simulink model "sgMdl_IO751_IO752_PROFINETSynchronous"  (R2024b)
settings: Solver=FixedStepAuto  StartTime=0.0  StopTime=inf  RelTol=1e-3  EnableMultiTasking=on
undefined symbols (not defined in the file): C
libraries: slrealtimeutilitieslib x26, simulink x3, speedgoatlib_IO751 x3, speedgoatlib_IO752 x3, speedgoatlib_interrupt x2
Description:
  | IO751 & IO752 - Synchronous PROFINET
settings Model: ModifiedByFormat=Speedgoat  Creator=Speedgoat  LastModifiedBy=Speedgoat
settings SolverCC: ConcurrentTasks=on  AlgebraicLoopSolver=TrustRegion  PositivePriorityOrder=on  AutoInsertRateTranBlk=on  InsertRTBMode=Never (minimum delay)
settings DataIOCC: SaveFormat=Array  SaveState=on  SignalLoggingName=logsOut
settings OptimizationCC: BlockReduction=off  BooleanDataType=off  OptimizeBlockIOStorage=off  BufferReuse=off  ReuseModelBlockBuffer=off  GlobalBufferReuse=off  ExpressionFolding=off  LocalBlockOutputs=off  InitFltsAndDblsToZero=on  OptimizeDataStoreBuffers=off  BusAssignmentInplaceUpdate=off
settings DebuggingCC: SaveWithParameterizedLinksMsg=none  UnderspecifiedInitializationDetection=Classic  MergeDetectMultiDrivingBlocksExec=none  CheckExecutionContextPreStartOutputMsg=on  SignalResolutionControl=TryResolveAllWithWarning  TasksWithSamePriorityMsg=none  UnconnectedInputMsg=warning  UnconnectedOutputMsg=warning  UnconnectedLineMsg=warning  SFUnexpectedBacktrackingDiag=warning  SFNoUnconditionalDefaultTransitionDiag=warning  SFExecutionAtInitializationDiag=none  ArithmeticOperatorsInVariantConditions=warning
settings HardwareCC: ProdBitPerLong=64  ProdLongLongMode=on  ProdHWDeviceType=Intel->x86-64 (Linux 64)
settings ModelReferenceCC: EnableRefExpFcnMdlSchedulingChecks=on  PropagateSignalLabelsOutOfModel=off
settings SFSimCC: SimUseLocalCustomCode=off  SimTargetLang=C++
settings RTWCC: Description=Speedgoat Real-Time Target Machine  SystemTargetFile=speedgoat.tlc  TemplateMakefile=slrealtime_default_tmf  RTWUseLocalCustomCode=off  Toolchain=Simulink Real-Time Toolchain  BuildConfiguration=Faster Runs  TargetLang=C++  GPUComputeCapability=3.5  DLArmComputeVersion=19.05
settings CodeAppCC: StateflowObjectComments=on
settings SimulinkRealTimeTargetCC: SubcomponentCodeInterfacePackaging=Reusable function  InstructionSetFMA=off  LogToMDFFile=off  SLRTFileLogMaxRuns=10
settings ConfigComp: CovMetricSettings=dw  CovSaveCumulativeToWorkspaceVar=on  CovSaveSingleToWorkspaceVar=on  CovExternalEMLEnable=off  CovSFcnEnable=off  CovBoundaryAbsTol=1.0e-5

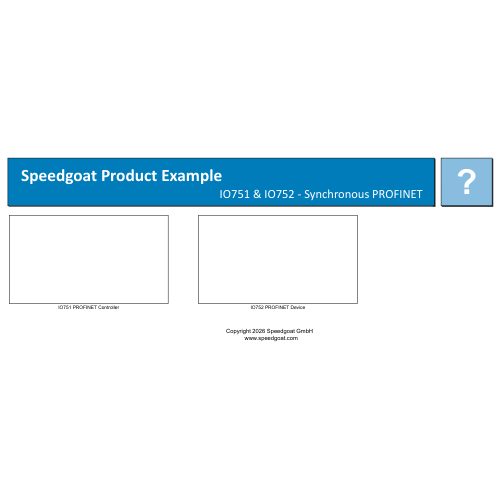
[thumbnail: Simulink's stored preview of the top-level diagram]
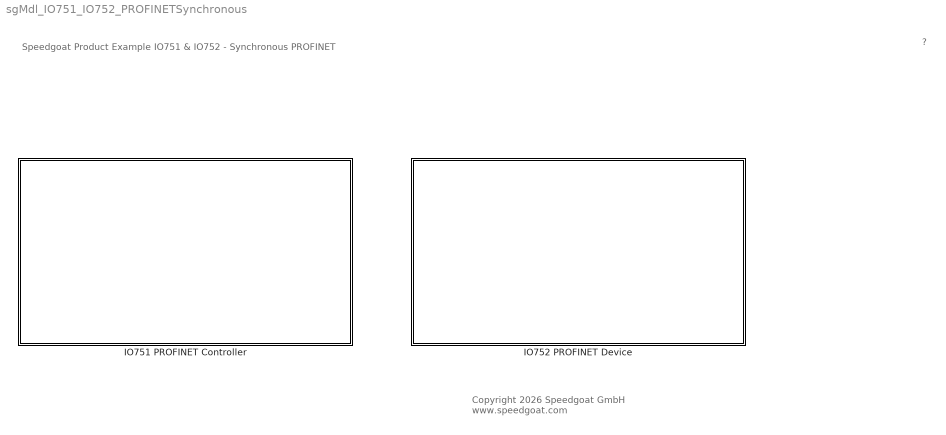
== system sgMdl_IO751_IO752_PROFINETSynchronous ==
  note: Speedgoat Product Example
      | IO751 & IO752 - Synchronous PROFINET
  note: ?
  note: Copyright 2026 Speedgoat GmbH
      |  www.speedgoat.com
  IO751 PROFINET Controller : Subsystem
  IO752 PROFINET Device : Subsystem

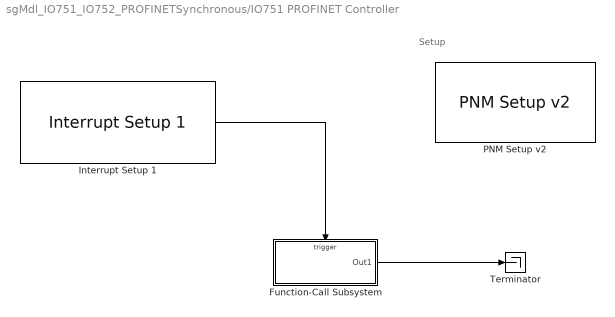
== system sgMdl_IO751_IO752_PROFINETSynchronous/IO751 PROFINET Controller ==
  note: Setup
  Function-Call Subsystem : Subsystem  TreatAsAtomicUnit=on
  Interrupt Setup 1 : speedgoatlib_interrupt/Interrupt Setup 1  parModuleTrigger=off  parPollingMode=off  parPriorityConf=High  parPriority=241  confStartFcn=IO75x_start_public  confStopFcn=IO75x_stop_public  confIsrFcn=IO75x_isr_public  confMapFcn=IO75x_map_public  confHookFile=io75x_int_hooks.c  confIrqNr=-1  confIsPolling=off  confModID=985345  confSelectedInt=Speedgoat IO75x interrupt  confSelectedId=1  confSelectedChannel=[]  confData=[]  confForcePollingMode=off
  "PNM Setup v2 " : speedgoatlib_IO751/PNM Setup v2   id=1  driveLetter=C:  configurationMode=Configuration file  mode=Polling mode  pciSlot=[9,15]  quantityOfAcyclicObjects=0  qtyMods=[1,0,0]  ConfigFile=which('IO751_IO752_Synchronous_m.nxd')  parOptAcyclic=off  protocol=IO751  firmware=PROFINET Controller
      settings: SourceProductName=IO751 PROFINET Controller
  Terminator : Terminator
  wires:
  Interrupt Setup 1/1 -> Function-Call Subsystem/Trigger
  Function-Call Subsystem/1(Out1) -> Terminator/1

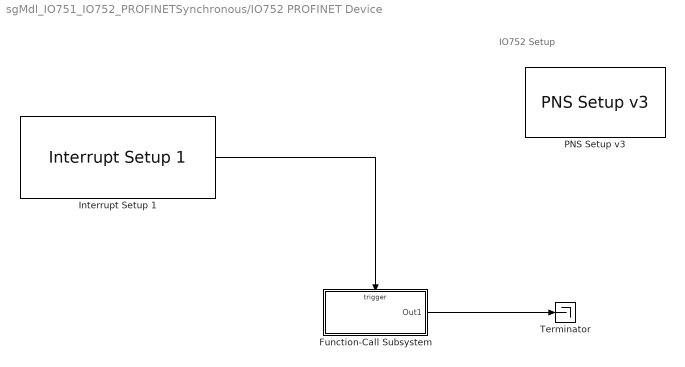
== system sgMdl_IO751_IO752_PROFINETSynchronous/IO752 PROFINET Device ==
  note: IO752 Setup
  Function-Call Subsystem : Subsystem  TreatAsAtomicUnit=on
  Interrupt Setup 1 : speedgoatlib_interrupt/Interrupt Setup 1  parModuleTrigger=off  parPollingMode=off  parPriorityConf=High  parPriority=241  confStartFcn=IO75x_start_public  confStopFcn=IO75x_stop_public  confIsrFcn=IO75x_isr_public  confMapFcn=IO75x_map_public  confHookFile=io75x_int_hooks.c  confIrqNr=-1  confIsPolling=off  confModID=919810  confSelectedInt=Speedgoat IO75x interrupt  confSelectedId=2  confSelectedChannel=[]  confData=[]  confForcePollingMode=off
  PNS Setup v3 : speedgoatlib_IO752/PNS Setup v3  id=2  PciSlot=[9,14]  StationName='cifxrepns'  BusStart=On model start  SystemRedundancy=off  RecordSuccess=on  GsdFile=[speedgoatroot, '\sg_blocks\cifx\eds\GSDML-V2.33-HILSCHER-CIFX RE PNS-20170919.xml']  VendorId=286  DeviceId=259  OptionalIdentity=off  DeviceType='cifxrepns'  OrderId='1250.1'  HwRev=2  SwRevPrefix='V'  SwRev=[3,0,0]  SerialNumber='0'  ModuleConfigTable="{ '0', '', 'CIFX RE/PNS V3.5.35 - V3.x', '8321', '', '', 'DIM 24', '', '', '0', '1', ''; '0', '1', '  CIFX RE/PNS V3.5.35 - V3.x', '8321', '8320', '', 'DIM 24', '1', '', '', '', ''; '0', '32768', '  PN-IO', '8321', '8321', '', 'DIM 24 Interfacesubmodule', '1', '', '', '', ''; '0', '32769', '  Port 1', '8321', '8322', '', 'DIM 24 Portsubmodule 1', '1', '', '', '', ''; '0', '32770', '  Port 2', '8321', '8323', '', 'DIM 24 Portsubmodule 2', '1', '', '', '', ''; '1', '', '4 Bytes Input', '8', '', '', '4byteinput', '0', '', '', '', ''; '1', '1', '  4 Bytes Input', '8', '7', '', '4byteinput', '1', '{\"Inputs\",[3],[4]}', '', '', ''; '2', '', '4 Bytes Output', '9', '', '', '4byteoutput', '0', '', '', '', ''; '2', '1', '  4 Bytes Output', '9', '8', '', '4byteoutput', '1', '', '{\"Outputs\",[3],[4]}', '', '' }"
      settings: SourceProductName=IO752 PROFINET Device
  Terminator : Terminator
  wires:
  Interrupt Setup 1/1 -> Function-Call Subsystem/Trigger
  Function-Call Subsystem/1(Out1) -> Terminator/1

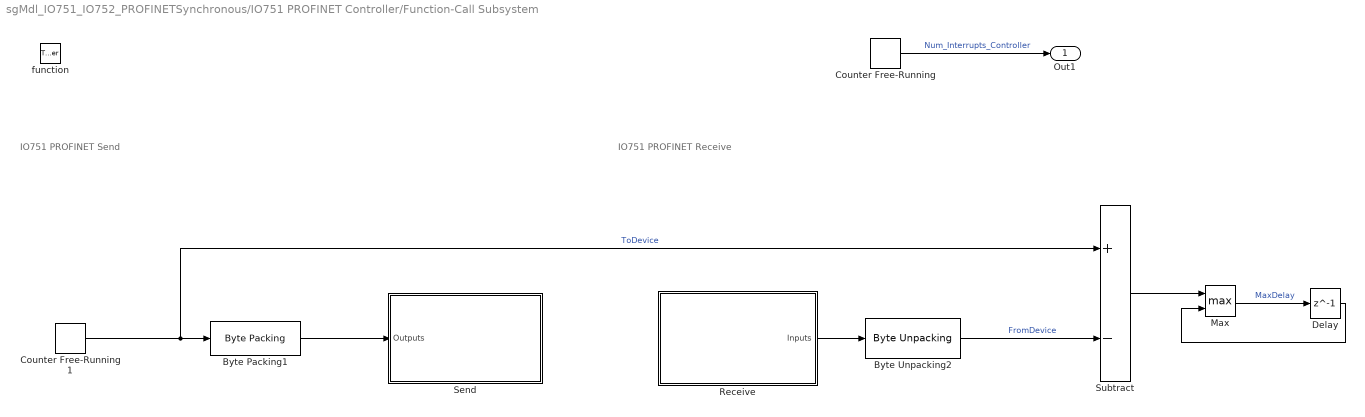
== system sgMdl_IO751_IO752_PROFINETSynchronous/IO751 PROFINET Controller/Function-Call Subsystem ==
  note: IO751 PROFINET Receive
  note: IO751 PROFINET Send
  function : TriggerPort  TriggerType=function-call  VariantControl=(inherit)
  Byte Packing1 : slrealtimeutilitieslib/Byte Packing  MaskPackedDataType=uint8  MaskUnpackedDataTypes={'uint32'}  MaskAlignment=1
  Byte Unpacking2 : slrealtimeutilitieslib/Byte Unpacking  MaskUnpackedDataTypes={'uint32'}  MaskUnpackedDataSizes={[1]}  MaskAlignment=1
  Counter Free-Running : simulink/Sources/Counter Free-Running  NumBits=16  tsamp=-1
  Counter Free-Running1 : simulink/Sources/Counter Free-Running  NumBits=32  tsamp=-1
  Delay : Delay  DelayLength=1
  Max : MinMax  Function=max  Inputs=2
  Receive : Subsystem
  Send : Subsystem
  Subtract : Sum  Inputs=+-
  Out1 : Outport
  wires:
  Counter Free-Running/1 -> Out1/1  "Num_Interrupts_Controller"
  Max/1 -> Delay/1  "MaxDelay"
  Delay/1 -> Max/2
  Counter Free-Running1/1 -> Subtract/1, Byte Packing1/1  "ToDevice"
  Subtract/1 -> Max/1
  Byte Packing1/1 -> Send/1(Outputs)
  Receive/1(Inputs) -> Byte Unpacking2/1
  Byte Unpacking2/1 -> Subtract/2  "FromDevice"

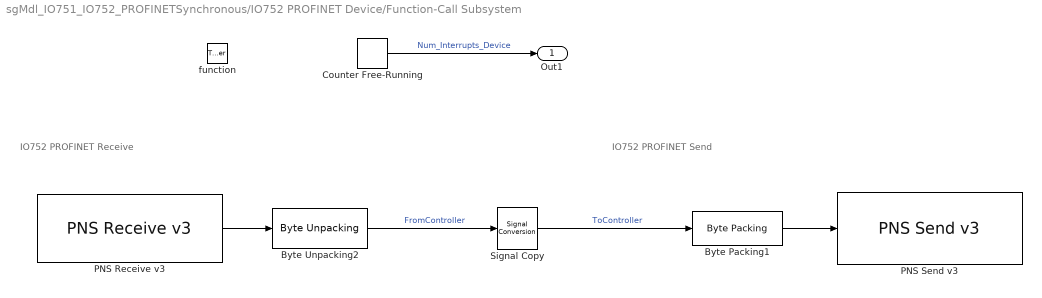
== system sgMdl_IO751_IO752_PROFINETSynchronous/IO752 PROFINET Device/Function-Call Subsystem ==
  note: IO752 PROFINET Receive
  note: IO752 PROFINET Send
  function : TriggerPort  TriggerType=function-call  VariantControl=(inherit)
  Byte Packing1 : slrealtimeutilitieslib/Byte Packing  MaskPackedDataType=uint8  MaskUnpackedDataTypes={'uint32'}  MaskAlignment=1
  Byte Unpacking2 : slrealtimeutilitieslib/Byte Unpacking  MaskUnpackedDataTypes={'uint32'}  MaskUnpackedDataSizes={[1]}  MaskAlignment=1
  Counter Free-Running : simulink/Sources/Counter Free-Running  NumBits=16  tsamp=-1
  PNS Receive v3 : speedgoatlib_IO752/PNS Receive v3  id=2  SampleTime=-1  DataLevel=Data Item  GroupDataItems=off  PortLabel1=off  PortLabel2=on  PortLabel3=off  PnModuleConfig="{ '0', '', 'CIFX RE/PNS V3.5.35 - V3.x', '8321', '', '', 'DIM 24', '', '', '0', '1', ''; '0', '1', '  CIFX RE/PNS V3.5.35 - V3.x', '8321', '8320', '', 'DIM 24', '1', '', '', '', ''; '0', '32768', '  PN-IO', '8321', '8321', '', 'DIM 24 Interfacesubmodule', '1', '', '', '', ''; '0', '32769', '  Port 1', '8321', '8322', '', 'DIM 24 Portsubmodule 1', '1', '', '', '', ''; '0', '32770', '  Port 2', '8321', '8323', '', 'DIM 24 Portsubmodule 2', '1', '', '', '', ''; '1', '', '4 Bytes Input', '8', '', '', '4byteinput', '0', '', '', '', ''; '1', '1', '  4 Bytes Input', '8', '7', '', '4byteinput', '1', '{\"Inputs\",[3],[4]}', '', '', ''; '2', '', '4 Bytes Output', '9', '', '', '4byteoutput', '0', '', '', '', ''; '2', '1', '  4 Bytes Output', '9', '8', '', '4byteoutput', '1', '', '{\"Outputs\",[3],[4]}', '', '' }"
      settings: SourceProductName=IO752 PROFINET Device
  PNS Send v3 : speedgoatlib_IO752/PNS Send v3  id=2  SampleTime=-1  DataLevel=Data Item  GroupDataItems=off  PortLabel1=off  PortLabel2=on  PortLabel3=off  PnModuleConfig="{ '0', '', 'CIFX RE/PNS V3.5.35 - V3.x', '8321', '', '', 'DIM 24', '', '', '0', '1', ''; '0', '1', '  CIFX RE/PNS V3.5.35 - V3.x', '8321', '8320', '', 'DIM 24', '1', '', '', '', ''; '0', '32768', '  PN-IO', '8321', '8321', '', 'DIM 24 Interfacesubmodule', '1', '', '', '', ''; '0', '32769', '  Port 1', '8321', '8322', '', 'DIM 24 Portsubmodule 1', '1', '', '', '', ''; '0', '32770', '  Port 2', '8321', '8323', '', 'DIM 24 Portsubmodule 2', '1', '', '', '', ''; '1', '', '4 Bytes Input', '8', '', '', '4byteinput', '0', '', '', '', ''; '1', '1', '  4 Bytes Input', '8', '7', '', '4byteinput', '1', '{\"Inputs\",[3],[4]}', '', '', ''; '2', '', '4 Bytes Output', '9', '', '', '4byteoutput', '0', '', '', '', ''; '2', '1', '  4 Bytes Output', '9', '8', '', '4byteoutput', '1', '', '{\"Outputs\",[3],[4]}', '', '' }"
      settings: SourceProductName=IO752 PROFINET Device
  Signal Copy : SignalConversion  OverrideOpt=off
  Out1 : Outport
  wires:
  PNS Receive v3/1 -> Byte Unpacking2/1
  Counter Free-Running/1 -> Out1/1  "Num_Interrupts_Device"
  Signal Copy/1 -> Byte Packing1/1  "ToController"
  Byte Unpacking2/1 -> Signal Copy/1  "FromController"
  Byte Packing1/1 -> PNS Send v3/1

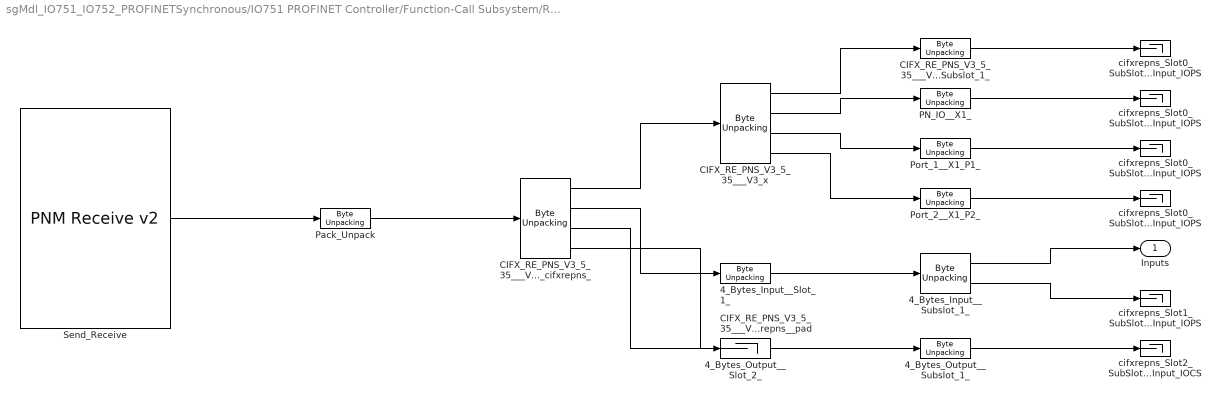
== system sgMdl_IO751_IO752_PROFINETSynchronous/IO751 PROFINET Controller/Function-Call Subsystem/Receive ==
  4_Bytes_Input__Slot_1_ : slrealtimeutilitieslib/Byte Unpacking  MaskUnpackedDataTypes={'uint8'}  MaskUnpackedDataSizes={[5]}  MaskAlignment=1
  4_Bytes_Input__Subslot_1_ : slrealtimeutilitieslib/Byte Unpacking  MaskUnpackedDataTypes={'uint8','uint8'}  MaskUnpackedDataSizes={[4],[1]}  MaskAlignment=1
  4_Bytes_Output__Slot_2_ : slrealtimeutilitieslib/Byte Unpacking  MaskUnpackedDataTypes={'uint8'}  MaskUnpackedDataSizes={[1]}  MaskAlignment=1
  4_Bytes_Output__Subslot_1_ : slrealtimeutilitieslib/Byte Unpacking  MaskUnpackedDataTypes={'uint8'}  MaskUnpackedDataSizes={[1]}  MaskAlignment=1
  CIFX_RE_PNS_V3_5_35___V3_x : slrealtimeutilitieslib/Byte Unpacking  MaskUnpackedDataTypes={'uint8','uint8','uint8','uint8'}  MaskUnpackedDataSizes={[1],[1],[1],[1]}  MaskAlignment=1
  CIFX_RE_PNS_V3_5_35___V3_x_CIFX_RE_PNS_V3_5_35___V3_x__cifxrepns_ : slrealtimeutilitieslib/Byte Unpacking  MaskUnpackedDataTypes={'uint8','uint8','uint8','uint8'}  MaskUnpackedDataSizes={[4],[5],[1],[2]}  MaskAlignment=1
  CIFX_RE_PNS_V3_5_35___V3_x_CIFX_RE_PNS_V3_5_35___V3_x__cifxrepns__pad : Terminator
  CIFX_RE_PNS_V3_5_35___V3_x__Subslot_1_ : slrealtimeutilitieslib/Byte Unpacking  MaskUnpackedDataTypes={'uint8'}  MaskUnpackedDataSizes={[1]}  MaskAlignment=1
  PN_IO__X1_ : slrealtimeutilitieslib/Byte Unpacking  MaskUnpackedDataTypes={'uint8'}  MaskUnpackedDataSizes={[1]}  MaskAlignment=1
  Pack_Unpack : slrealtimeutilitieslib/Byte Unpacking  MaskUnpackedDataTypes={'uint8'}  MaskUnpackedDataSizes={[12]}  MaskAlignment=1
  Port_1__X1_P1_ : slrealtimeutilitieslib/Byte Unpacking  MaskUnpackedDataTypes={'uint8'}  MaskUnpackedDataSizes={[1]}  MaskAlignment=1
  Port_2__X1_P2_ : slrealtimeutilitieslib/Byte Unpacking  MaskUnpackedDataTypes={'uint8'}  MaskUnpackedDataSizes={[1]}  MaskAlignment=1
  Send_Receive : speedgoatlib_IO751/PNM Receive v2   id=1  portType=1 port with n element vector of type UINT8  inputOutput=12  sampleTime=-1
      settings: SourceProductName=IO751 PROFINET Controller
  cifxrepns_Slot0_SubSlot1_Input_IOPS : Terminator
  cifxrepns_Slot0_SubSlot32768_Input_IOPS : Terminator
  cifxrepns_Slot0_SubSlot32769_Input_IOPS : Terminator
  cifxrepns_Slot0_SubSlot32770_Input_IOPS : Terminator
  cifxrepns_Slot1_SubSlot1_Input_IOPS : Terminator
  cifxrepns_Slot2_SubSlot1_Input_IOCS : Terminator
  Inputs : Outport  OutDataTypeStr=uint8  PortDimensions=4
  wires:
  CIFX_RE_PNS_V3_5_35___V3_x__Subslot_1_/1 -> cifxrepns_Slot0_SubSlot1_Input_IOPS/1
  PN_IO__X1_/1 -> cifxrepns_Slot0_SubSlot32768_Input_IOPS/1
  Port_1__X1_P1_/1 -> cifxrepns_Slot0_SubSlot32769_Input_IOPS/1
  Port_2__X1_P2_/1 -> cifxrepns_Slot0_SubSlot32770_Input_IOPS/1
  CIFX_RE_PNS_V3_5_35___V3_x/1 -> CIFX_RE_PNS_V3_5_35___V3_x__Subslot_1_/1
  CIFX_RE_PNS_V3_5_35___V3_x/2 -> PN_IO__X1_/1
  CIFX_RE_PNS_V3_5_35___V3_x/3 -> Port_1__X1_P1_/1
  CIFX_RE_PNS_V3_5_35___V3_x/4 -> Port_2__X1_P2_/1
  4_Bytes_Input__Subslot_1_/1 -> Inputs/1
  4_Bytes_Input__Subslot_1_/2 -> cifxrepns_Slot1_SubSlot1_Input_IOPS/1
  4_Bytes_Input__Slot_1_/1 -> 4_Bytes_Input__Subslot_1_/1
  4_Bytes_Output__Subslot_1_/1 -> cifxrepns_Slot2_SubSlot1_Input_IOCS/1
  4_Bytes_Output__Slot_2_/1 -> 4_Bytes_Output__Subslot_1_/1
  CIFX_RE_PNS_V3_5_35___V3_x_CIFX_RE_PNS_V3_5_35___V3_x__cifxrepns_/1 -> CIFX_RE_PNS_V3_5_35___V3_x/1
  CIFX_RE_PNS_V3_5_35___V3_x_CIFX_RE_PNS_V3_5_35___V3_x__cifxrepns_/2 -> 4_Bytes_Input__Slot_1_/1
  CIFX_RE_PNS_V3_5_35___V3_x_CIFX_RE_PNS_V3_5_35___V3_x__cifxrepns_/3 -> 4_Bytes_Output__Slot_2_/1
  CIFX_RE_PNS_V3_5_35___V3_x_CIFX_RE_PNS_V3_5_35___V3_x__cifxrepns_/4 -> CIFX_RE_PNS_V3_5_35___V3_x_CIFX_RE_PNS_V3_5_35___V3_x__cifxrepns__pad/1
  Pack_Unpack/1 -> CIFX_RE_PNS_V3_5_35___V3_x_CIFX_RE_PNS_V3_5_35___V3_x__cifxrepns_/1
  Send_Receive/1 -> Pack_Unpack/1

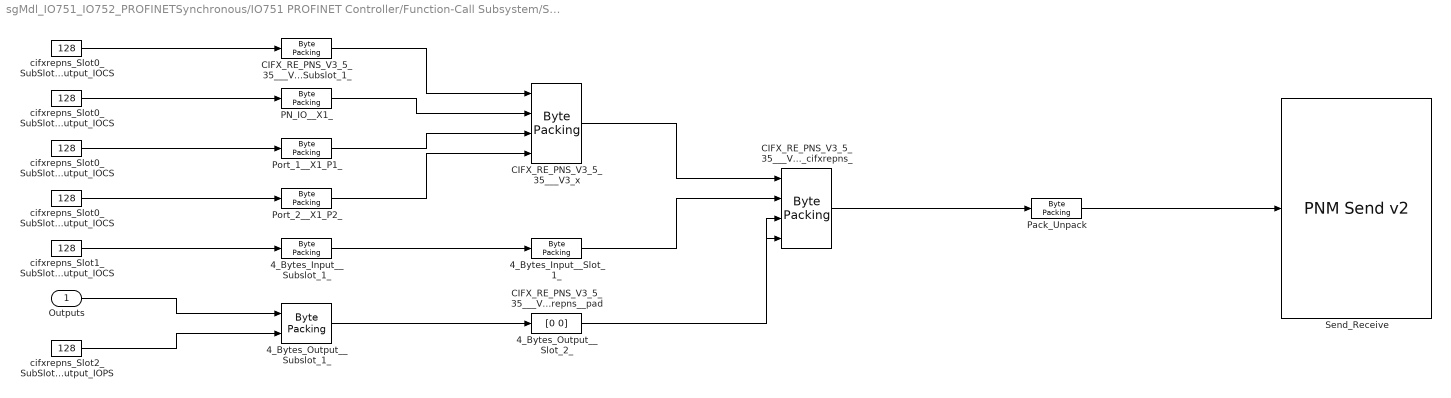
== system sgMdl_IO751_IO752_PROFINETSynchronous/IO751 PROFINET Controller/Function-Call Subsystem/Send ==
  Outputs : Inport  OutDataTypeStr=uint8  PortDimensions=4
  4_Bytes_Input__Slot_1_ : slrealtimeutilitieslib/Byte Packing  MaskPackedDataType=uint8  MaskUnpackedDataTypes={'uint8'}  MaskAlignment=1
  4_Bytes_Input__Subslot_1_ : slrealtimeutilitieslib/Byte Packing  MaskPackedDataType=uint8  MaskUnpackedDataTypes={'uint8'}  MaskAlignment=1
  4_Bytes_Output__Slot_2_ : slrealtimeutilitieslib/Byte Packing  MaskPackedDataType=uint8  MaskUnpackedDataTypes={'uint8'}  MaskAlignment=1
  4_Bytes_Output__Subslot_1_ : slrealtimeutilitieslib/Byte Packing  MaskPackedDataType=uint8  MaskUnpackedDataTypes={'uint8','uint8'}  MaskAlignment=1
  CIFX_RE_PNS_V3_5_35___V3_x : slrealtimeutilitieslib/Byte Packing  MaskPackedDataType=uint8  MaskUnpackedDataTypes={'uint8','uint8','uint8','uint8'}  MaskAlignment=1
  CIFX_RE_PNS_V3_5_35___V3_x_CIFX_RE_PNS_V3_5_35___V3_x__cifxrepns_ : slrealtimeutilitieslib/Byte Packing  MaskPackedDataType=uint8  MaskUnpackedDataTypes={'uint8','uint8','uint8','uint8'}  MaskAlignment=1
  CIFX_RE_PNS_V3_5_35___V3_x_CIFX_RE_PNS_V3_5_35___V3_x__cifxrepns__pad : Constant  Value=[0 0]  OutDataTypeStr=uint8
  CIFX_RE_PNS_V3_5_35___V3_x__Subslot_1_ : slrealtimeutilitieslib/Byte Packing  MaskPackedDataType=uint8  MaskUnpackedDataTypes={'uint8'}  MaskAlignment=1
  PN_IO__X1_ : slrealtimeutilitieslib/Byte Packing  MaskPackedDataType=uint8  MaskUnpackedDataTypes={'uint8'}  MaskAlignment=1
  Pack_Unpack : slrealtimeutilitieslib/Byte Packing  MaskPackedDataType=uint8  MaskUnpackedDataTypes={'uint8'}  MaskAlignment=1
  Port_1__X1_P1_ : slrealtimeutilitieslib/Byte Packing  MaskPackedDataType=uint8  MaskUnpackedDataTypes={'uint8'}  MaskAlignment=1
  Port_2__X1_P2_ : slrealtimeutilitieslib/Byte Packing  MaskPackedDataType=uint8  MaskUnpackedDataTypes={'uint8'}  MaskAlignment=1
  Send_Receive : speedgoatlib_IO751/PNM Send v2   id=1  portType=1 port with n element vector of type UINT8  inputOutput=12  sampleTime=-1
      settings: SourceProductName=IO751 PROFINET Controller
  cifxrepns_Slot0_SubSlot1_Output_IOCS : Constant  Value=128  OutDataTypeStr=uint8
  cifxrepns_Slot0_SubSlot32768_Output_IOCS : Constant  Value=128  OutDataTypeStr=uint8
  cifxrepns_Slot0_SubSlot32769_Output_IOCS : Constant  Value=128  OutDataTypeStr=uint8
  cifxrepns_Slot0_SubSlot32770_Output_IOCS : Constant  Value=128  OutDataTypeStr=uint8
  cifxrepns_Slot1_SubSlot1_Output_IOCS : Constant  Value=128  OutDataTypeStr=uint8
  cifxrepns_Slot2_SubSlot1_Output_IOPS : Constant  Value=128  OutDataTypeStr=uint8
  wires:
  cifxrepns_Slot0_SubSlot1_Output_IOCS/1 -> CIFX_RE_PNS_V3_5_35___V3_x__Subslot_1_/1
  cifxrepns_Slot0_SubSlot32768_Output_IOCS/1 -> PN_IO__X1_/1
  cifxrepns_Slot0_SubSlot32769_Output_IOCS/1 -> Port_1__X1_P1_/1
  cifxrepns_Slot0_SubSlot32770_Output_IOCS/1 -> Port_2__X1_P2_/1
  CIFX_RE_PNS_V3_5_35___V3_x__Subslot_1_/1 -> CIFX_RE_PNS_V3_5_35___V3_x/1
  PN_IO__X1_/1 -> CIFX_RE_PNS_V3_5_35___V3_x/2
  Port_1__X1_P1_/1 -> CIFX_RE_PNS_V3_5_35___V3_x/3
  Port_2__X1_P2_/1 -> CIFX_RE_PNS_V3_5_35___V3_x/4
  cifxrepns_Slot1_SubSlot1_Output_IOCS/1 -> 4_Bytes_Input__Subslot_1_/1
  4_Bytes_Input__Subslot_1_/1 -> 4_Bytes_Input__Slot_1_/1
  Outputs/1 -> 4_Bytes_Output__Subslot_1_/1
  cifxrepns_Slot2_SubSlot1_Output_IOPS/1 -> 4_Bytes_Output__Subslot_1_/2
  4_Bytes_Output__Subslot_1_/1 -> 4_Bytes_Output__Slot_2_/1
  CIFX_RE_PNS_V3_5_35___V3_x/1 -> CIFX_RE_PNS_V3_5_35___V3_x_CIFX_RE_PNS_V3_5_35___V3_x__cifxrepns_/1
  4_Bytes_Input__Slot_1_/1 -> CIFX_RE_PNS_V3_5_35___V3_x_CIFX_RE_PNS_V3_5_35___V3_x__cifxrepns_/2
  4_Bytes_Output__Slot_2_/1 -> CIFX_RE_PNS_V3_5_35___V3_x_CIFX_RE_PNS_V3_5_35___V3_x__cifxrepns_/3
  CIFX_RE_PNS_V3_5_35___V3_x_CIFX_RE_PNS_V3_5_35___V3_x__cifxrepns__pad/1 -> CIFX_RE_PNS_V3_5_35___V3_x_CIFX_RE_PNS_V3_5_35___V3_x__cifxrepns_/4
  CIFX_RE_PNS_V3_5_35___V3_x_CIFX_RE_PNS_V3_5_35___V3_x__cifxrepns_/1 -> Pack_Unpack/1
  Pack_Unpack/1 -> Send_Receive/1
